simulink model "controlador_modelo_bike"  (R2023a)
settings: configuration reference "Configuration" (kept outside this file)
libraries: simulink_extras x1, drivingvehiclecontroller x1
settings Model: DataDictionary=controlador_modelo_bike.sldd  Creator=thailon  LastModifiedBy=thailon
settings ConfigSetRef: SourceName=Configuration

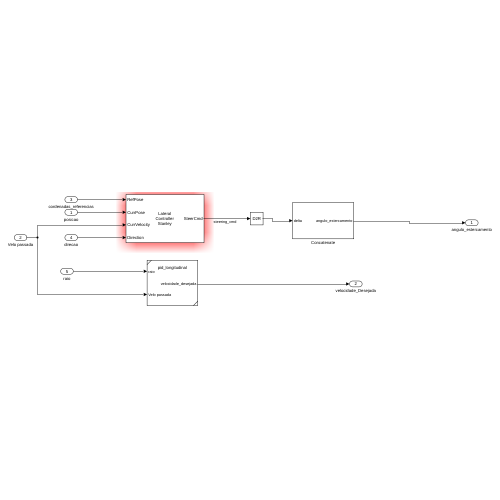
[thumbnail: Simulink's stored preview of the top-level diagram]
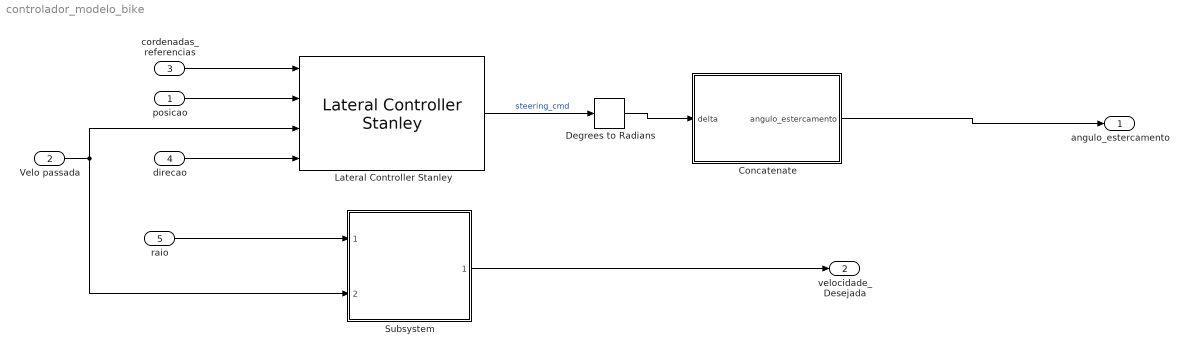
== system controlador_modelo_bike ==
  posicao : Inport
  Velo passada : Inport  Port=2
  cordenadas_referencias : Inport  Port=3
  direcao : Inport  Port=4
  raio : Inport  Port=5
  Concatenate : Subsystem
  Degrees to Radians : simulink_extras/Transformations/Degrees to Radians
  Lateral Controller Stanley : drivingvehiclecontroller/Lateral Controller Stanley  ModelType=Dynamic bicycle model  PositionGainF=stanley_kpfw  PositionGainR=stanley_kprv  YawRateGain=1  DelayGain=0.2  VehicleMass=230  Lf=1.4  Lr=1.6  TireStiffness=12e3  Wheelbase=wheelbase  MaxSteeringAngle=max_steering_angle
  Subsystem : Subsystem  ReferencedSubsystem=pid_longitudinal
  angulo_estercamento : Outport
  velocidade_Desejada : Outport  Port=2
  wires:
  Velo passada/1 -> Subsystem/2, Lateral Controller Stanley/3
  posicao/1 -> Lateral Controller Stanley/2
  Concatenate/1(angulo_estercamento) -> angulo_estercamento/1
  Degrees to Radians/1 -> Concatenate/1(delta)
  direcao/1 -> Lateral Controller Stanley/4
  cordenadas_referencias/1 -> Lateral Controller Stanley/1
  Lateral Controller Stanley/1 -> Degrees to Radians/1  "steering_cmd"
  raio/1 -> Subsystem/1
  Subsystem/1 -> velocidade_Desejada/1

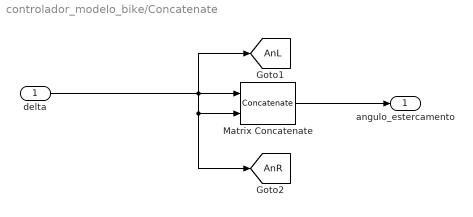
== system controlador_modelo_bike/Concatenate ==
  delta : Inport
  Matrix Concatenate : Concatenate
  angulo_estercamento : Outport  VectorParamsAs1DForOutWhenUnconnected=off
  tag scope: AnL=global, AnR=global
  wires:
  delta/1 -> Matrix Concatenate/1, Matrix Concatenate/2, [AnR], [AnL]
  Matrix Concatenate/1 -> angulo_estercamento/1
